simulink model "Pulse6Rectifier"  (R2023b)
settings: Solver=VariableStepAuto  StartTime=0.0  StopTime=0.1  RelTol=1e-3
libraries: spsCurrentMeasurementLib x8, spsDiodeLib x6, spsVoltageMeasurementLib x4, spsACVoltageSourceLib x3, spsGroundLib x1, spsSeriesRLCBranchLib x1, spspowerguiLib x1
settings Model: Creator=HP  LastModifiedBy=HP
settings DataIOCC: Refine=10

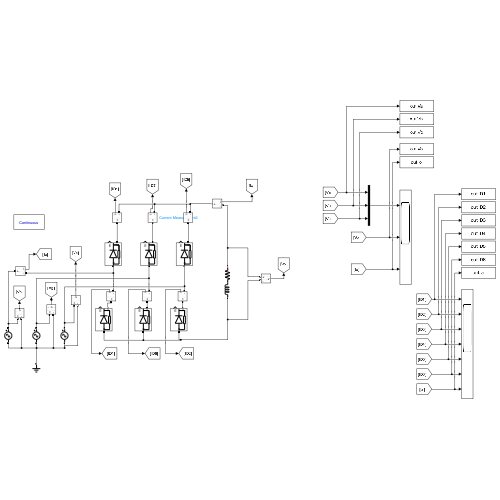
[thumbnail: Simulink's stored preview of the top-level diagram]
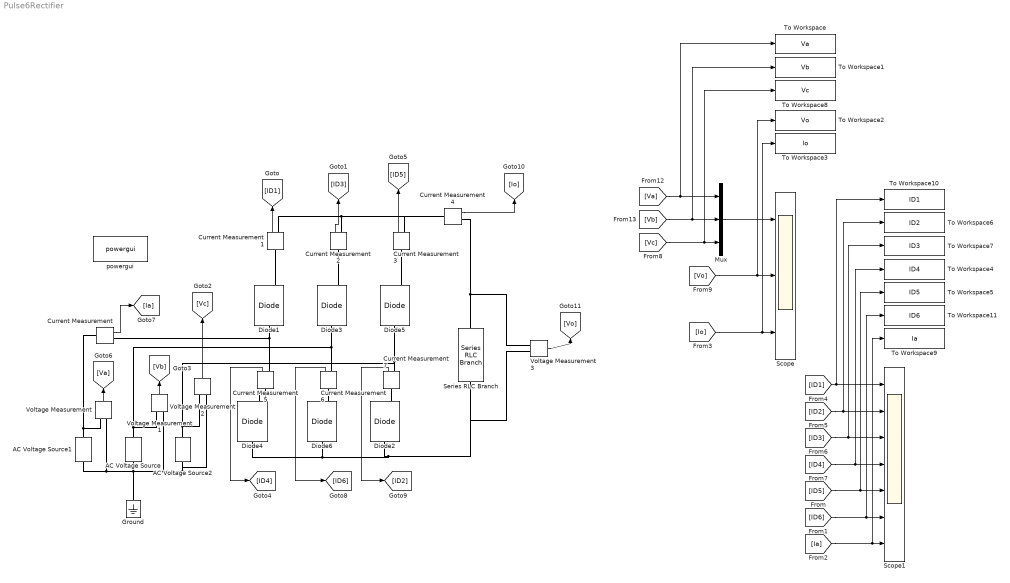
== system Pulse6Rectifier ==
  AC Voltage Source : spsACVoltageSourceLib/AC Voltage Source  Amplitude=480*sqrt(2)/sqrt(3)  Phase=-120  Frequency=60  SampleTime=0  Measurements=None  BusType=swing  Pref=10e3  Qref=0  Qmin=-inf  Qmax=+inf
  AC Voltage Source1 : spsACVoltageSourceLib/AC Voltage Source  Amplitude=480*sqrt(2)/sqrt(3)  Phase=0  Frequency=60  SampleTime=0  Measurements=None  BusType=swing  Pref=10e3  Qref=0  Qmin=-inf  Qmax=+inf
  AC Voltage Source2 : spsACVoltageSourceLib/AC Voltage Source  Amplitude=480*sqrt(2)/sqrt(3)  Phase=120  Frequency=60  SampleTime=0  Measurements=None  BusType=swing  Pref=10e3  Qref=0  Qmin=-inf  Qmax=+inf
  Current Measurement{,1..7} (8 alike) : spsCurrentMeasurementLib/Current Measurement  PhasorSimulation=off  OutputType=Complex  PSBequivalent=0
  Diode{1..6} (6 alike) : spsDiodeLib/Diode  Ron=0.001  Lon=0  Vf=0.8  IC=0  UseSnubber=0  Rs=500  Cs=250e-9  Measurements=on
  Ground : spsGroundLib/Ground  LConnTagsString=a
  Mux : Mux  Inputs=3
  Scope : Scope  NumInputPorts=3
  Scope1 : Scope  NumInputPorts=7
  Series RLC Branch : spsSeriesRLCBranchLib/Series RLC Branch  LConnTagsString=__new0  RConnTagsString=__new0  BranchType=RL  Resistance=11.08  Inductance=0.0224  SetiL0=off  InitialCurrent=0  Capacitance=0  Setx0=off  InitialVoltage=0  Measurements=None
  To Workspace : ToWorkspace  VariableName=Va  SaveFormat=Timeseries  SampleTime=-1
  To Workspace1 : ToWorkspace  VariableName=Vb  SaveFormat=Timeseries  SampleTime=-1
  To Workspace10 : ToWorkspace  VariableName=ID1  SaveFormat=Timeseries  SampleTime=-1
  To Workspace11 : ToWorkspace  VariableName=ID6  SaveFormat=Timeseries  SampleTime=-1
  To Workspace2 : ToWorkspace  VariableName=Vo  SaveFormat=Timeseries  SampleTime=-1
  To Workspace3 : ToWorkspace  VariableName=Io  SaveFormat=Timeseries  SampleTime=-1
  To Workspace4 : ToWorkspace  VariableName=ID4  SaveFormat=Timeseries  SampleTime=-1
  To Workspace5 : ToWorkspace  VariableName=ID5  SaveFormat=Timeseries  SampleTime=-1
  To Workspace6 : ToWorkspace  VariableName=ID2  SaveFormat=Timeseries  SampleTime=-1
  To Workspace7 : ToWorkspace  VariableName=ID3  SaveFormat=Timeseries  SampleTime=-1
  To Workspace8 : ToWorkspace  VariableName=Vc  SaveFormat=Timeseries  SampleTime=-1
  To Workspace9 : ToWorkspace  VariableName=Ia  SaveFormat=Timeseries  SampleTime=-1
  Voltage Measurement{,1..3} (4 alike) : spsVoltageMeasurementLib/Voltage Measurement  PhasorSimulation=off  OutputType=Complex  PSBequivalent=0
  powergui : spspowerguiLib/powergui  Priority=1  SimulationMode=Continuous  SampleTime=50e-6  frequency=60  Iterations=50  frequencyindice=60  Pbase=100e6  ErrMax=1e-4  UnitsV=kV  UnitsW=MW  buscounter=0  FunctionMessages=off  echomessages=off  EnableUseOfTLC=off  CurrentSourceSwitches=off  DisableSnubberDevices=off  DisableRonSwitches=off  DisableVfSwitches=off  DisplayEquations=off  AutomaticDiscreteSolvers=off  SolverType=Tustin/Backward Euler (TBE)  Interpol=off  ExternalGateDelay=off  methode=off  Ts=100  x0status=blocks  SPID=on  SwTol=0  HookPort=off  NonlinearTolerance=1e-4  nMaxIteration=100  ContinueOnMaxIteration=off  RestoreLinks=warning  ResistiveCurrentMeasurement=off  Frange=[0:2:500]  Ylog=off  Xlog=on  ShowGrid=off  save=off  variable=ZData  structure=0  ZoomFFT=off  StartTime=0.0  cycles=1  DisplayStyle=1  fundamental=60  FreqAxis=off  MaxFrequency=1000  frequencyindicesteady=1  RmsSteady=1  display=off
  wires:
  Current Measurement/1 -> [Ia]
  Voltage Measurement/1 -> [Va]
  Voltage Measurement1/1 -> [Vb]
  Voltage Measurement2/1 -> [Vc]
  Current Measurement1/1 -> [ID1]
  Current Measurement2/1 -> [ID3]
  Current Measurement3/1 -> [ID5]
  Current Measurement4/1 -> [Io]
  Voltage Measurement3/1 -> [Vo]
  [Vb] -> To Workspace1/1, Mux/2
  [Va] -> To Workspace/1, Mux/1
  [Vc] -> To Workspace8/1, Mux/3
  Mux/1 -> Scope/1
  [Vo] -> To Workspace2/1, Scope/2
  [Io] -> To Workspace3/1, Scope/3
  [ID1] -> To Workspace10/1, Scope1/1
  [ID2] -> To Workspace6/1, Scope1/2
  [ID3] -> To Workspace7/1, Scope1/3
  [ID4] -> To Workspace4/1, Scope1/4
  [ID5] -> To Workspace5/1, Scope1/5
  [ID6] -> To Workspace11/1, Scope1/6
  [Ia] -> To Workspace9/1, Scope1/7
  Current Measurement5/1 -> [ID4]
  Current Measurement6/1 -> [ID6]
  Current Measurement7/1 -> [ID2]
  connections:
  Current Measurement1/RConn1 -- Current Measurement3/RConn1 -- Current Measurement4/LConn1 -- Current Measurement2/RConn1
  Diode3/LConn1 -- Current Measurement6/RConn1 -- Voltage Measurement1/LConn1 -- AC Voltage Source/RConn1
  Diode5/LConn1 -- Voltage Measurement2/LConn1 -- AC Voltage Source2/RConn1 -- Current Measurement7/RConn1
  Voltage Measurement/LConn1 -- Current Measurement/LConn1 -- AC Voltage Source1/RConn1
  Diode4/LConn1 -- Series RLC Branch/RConn1 -- Voltage Measurement3/LConn2 -- Diode2/LConn1 -- Diode6/LConn1
  AC Voltage Source2/LConn1 -- Voltage Measurement2/LConn2 -- Voltage Measurement1/LConn2 -- Ground/LConn1 -- AC Voltage Source/LConn1 -- AC Voltage Source1/LConn1 -- Voltage Measurement/LConn2
  Current Measurement/RConn1 -- Diode1/LConn1 -- Current Measurement5/RConn1
  Current Measurement1/LConn1 -- Diode1/RConn1
  Current Measurement2/LConn1 -- Diode3/RConn1
  Voltage Measurement3/LConn1 -- Current Measurement4/RConn1 -- Series RLC Branch/LConn1
  Diode5/RConn1 -- Current Measurement3/LConn1
  Current Measurement5/LConn1 -- Diode4/RConn1
  Diode2/RConn1 -- Current Measurement7/LConn1
  Diode6/RConn1 -- Current Measurement6/LConn1
